simulink model "PT"  (R2025b)
settings: Solver=FixedStepAuto  StartTime=0.0  StopTime=Sim_Duration  FixedStep=1/500  RelTol=1e-3
values from neighbouring files (symbols this model uses):
  Kv_1_max = 1.5    [EReg_N2O_Simulink_Init.m]    (also in EReg_Tank_Drain_Init.m = 1; EReg_Tank_Drain_N2O_Sim.m = params.Kv_1_max)
  P_1_0 = 300e5    (= 30000000)    [EReg_N2O_Simulink_Init.m]    (also in EReg_Tank_Drain_Init.m; EReg_Tank_Drain_N2O_Sim.m = params.P_1_0)
libraries: simulink x1
settings Model: Creator=marti  LastModifiedBy=esthe
settings DataIOCC: SaveOutput=off  SaveTime=off
settings OptimizationCC: ReuseModelBlockBuffer=off
settings ModelReferenceCC: ModelReferenceMinAlgLoopOccurrences=on
settings RTWCC: GPUComputeCapability=3.5
settings GRTTargetCC: CombineOutputUpdateFcns=off

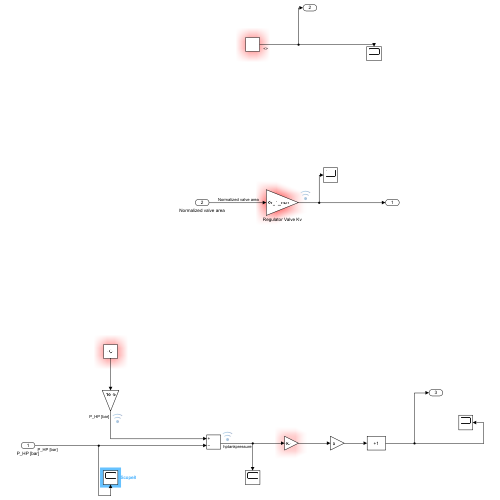
[thumbnail: Simulink's stored preview of the top-level diagram]
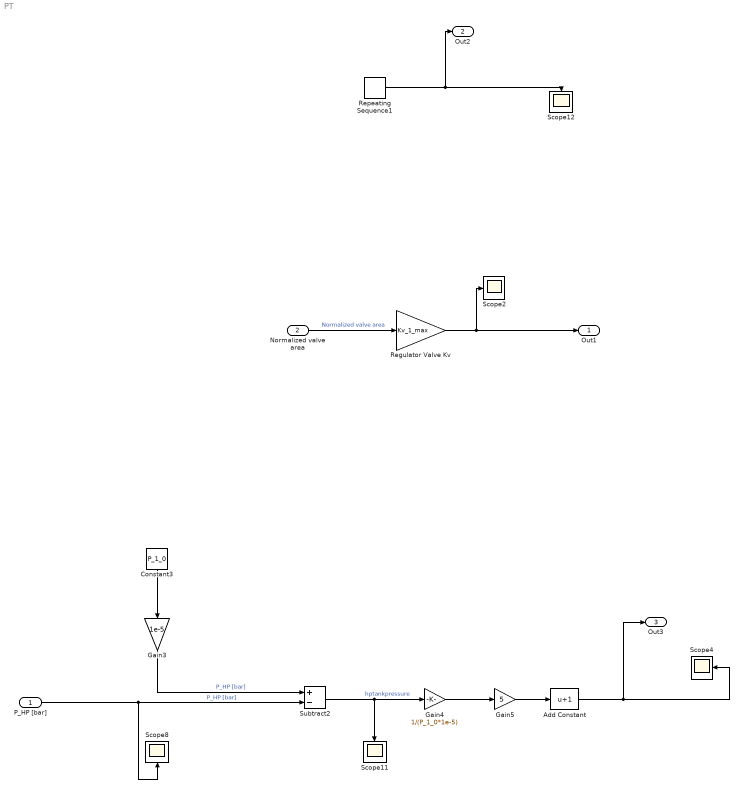
== system PT ==
  P_HP [bar] : Inport  OutDataTypeStr=double  PortDimensions=1  SampleTime=0
  Normalized valve area : Inport  Port=2  OutDataTypeStr=double  PortDimensions=1  SampleTime=0
  Add Constant : Bias  Bias=1  SaturateOnIntegerOverflow=off
  Constant3 : Constant  Value=P_1_0
  Gain3 : Gain  Gain=1e-5
  Gain4 : Gain  Gain=1/(P_1_0*1e-5)
  Gain5 : Gain  Gain=5
  Regulator Valve Kv : Gain  Gain=Kv_1_max
  Repeating Sequence1 : simulink/Sources/Repeating Sequence  rep_seq_t=time  rep_seq_y=run_valve_setpoint
  Scope{2,4,8,11..12} (5 alike) : Scope
      Scope11 settings: ActiveDisplayYMinimum=-7.98984  ActiveDisplayYMaximum=71.90855
      Scope12 settings: ActiveDisplayYMinimum=-0.125  ActiveDisplayYMaximum=1.125  DataLoggingVariableName=ScopeData2
      Scope2 settings: ActiveDisplayYMinimum=-0.0196  ActiveDisplayYMaximum=0.17636  DataLoggingVariableName=ScopeData3
      Scope4 settings: ActiveDisplayYMinimum=0.86684  ActiveDisplayYMaximum=2.19848
      Scope8 settings: ActiveDisplayYMinimum=229.43787  ActiveDisplayYMaximum=307.84024  DataLoggingVariableName=ScopeData4
  Subtract2 : Sum  Inputs=+-
  Out1 : Outport  OutDataTypeStr=double  PortDimensions=1  SampleTime=0
  Out2 : Outport  Port=2  OutDataTypeStr=double  PortDimensions=1  SampleTime=0
  Out3 : Outport  Port=3  OutDataTypeStr=double  PortDimensions=1  SampleTime=0
  wires:
  Gain4/1 -> Gain5/1
  Gain3/1 -> Subtract2/1  "P_HP [bar]"
  Normalized valve area/1 -> Regulator Valve Kv/1  "Normalized valve area"
  Add Constant/1 -> Out3/1, Scope4/1
  P_HP [bar]/1 -> Scope8/1, Subtract2/2  "P_HP [bar]"
  Gain5/1 -> Add Constant/1
  Regulator Valve Kv/1 -> Out1/1, Scope2/1
  Constant3/1 -> Gain3/1
  Repeating Sequence1/1 -> Scope12/1, Out2/1
  Subtract2/1 -> Gain4/1, Scope11/1  "hptankpressure"
